simulink model "power_surgnetwork"  (Simulink 6.0)
settings: Solver=ode15s  SolverMode=SingleTasking  StartTime=0.0  StopTime=0.2  RelTol=1e-3  AbsTol=1e-2
libraries: powerlib x21
settings Model: Creator=patrice  LastModifiedBy=batserve  ExtModeTrigMode=oneshot  ExtModeArmWhenConnect=off  ExtModeAutoUpdateStatusClock=off
settings DataIOCC: LimitDataPoints=off  SignalLoggingName=sigsOut
settings OptimizationCC: BlockReduction=off  BooleanDataType=off
settings DebuggingCC: AlgebraicLoopMsg=none  CheckExecutionContextPreStartOutputMsg=on  CheckExecutionContextRuntimeOutputMsg=on  SolverPrmCheckMsg=none
settings HardwareCC: TargetUnknown=on
settings RTWCC: TemplateMakefile=grt_unix.tmf

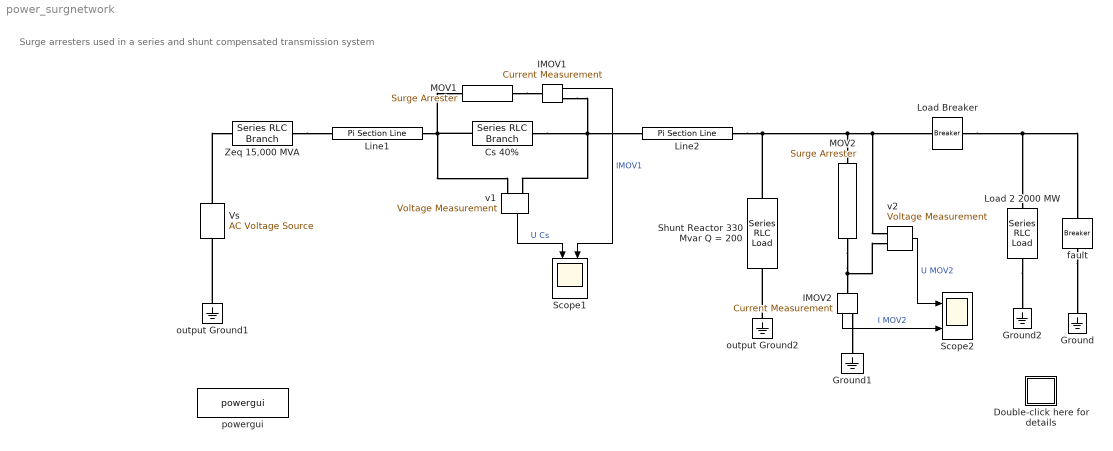
== system power_surgnetwork ==
  note: Surge arresters used in  a series and shunt  compensated
      | transmission system
  Cs 40% : powerlib/Elements/Series RLC Branch  PhysicalDomain=powersysdomain  SubClassName=unknown  LeftPortType=p1  RightPortType=p1  LConnTagsString=__new0  RConnTagsString=__new0  Resistance=0  Inductance=0  Capacitance=101.4e-6  Measurements=None
  Double-click here for details : Subsystem
      mask Display: disp('?')
  Ground : powerlib/Elements/Ground  Orientation=down  PhysicalDomain=powersysdomain  SubClassName=unknown  LeftPortType=p1  RightPortType=p1  LConnTagsString=a
  Ground1 : powerlib/Elements/Ground  Orientation=down  PhysicalDomain=powersysdomain  SubClassName=unknown  LeftPortType=p1  RightPortType=p1  LConnTagsString=a
  Ground2 : powerlib/Elements/Ground  Orientation=down  PhysicalDomain=powersysdomain  SubClassName=unknown  LeftPortType=p1  RightPortType=p1  LConnTagsString=a
  IMOV1 : powerlib/Measurements/Current Measurement  Tag=PoWeRsYsTeMmEaSuReMeNt  PhasorSimulation=off  OutputType=Magnitude  PSBequivalent=0
  IMOV2 : powerlib/Measurements/Current Measurement  Tag=PoWeRsYsTeMmEaSuReMeNt  Orientation=down  PhasorSimulation=off  OutputType=Magnitude  PSBequivalent=0
  Line1 : powerlib/Elements/Pi Section Line  PhysicalDomain=powersysdomain  SubClassName=unknown  LeftPortType=p1  RightPortType=p1  LConnTagsString=__new0  RConnTagsString=__new0  Frequency=60  Resistance=0.011  Inductance=0.8674e-3  Capacitance=13.41e-9  Length=100  PiSections=2  Measurements=None
      settings: AttributesFormatString=\n
  Line2 : powerlib/Elements/Pi Section Line  PhysicalDomain=powersysdomain  SubClassName=unknown  LeftPortType=p1  RightPortType=p1  LConnTagsString=__new0  RConnTagsString=__new0  Frequency=60  Resistance=0.011  Inductance=0.8674e-3  Capacitance=13.41e-9  Length=100  PiSections=2  Measurements=None
      settings: AttributesFormatString=\n
  Load 2 2000 MW : powerlib/Elements/Series RLC Load  Orientation=down  PhysicalDomain=powersysdomain  SubClassName=unknown  LeftPortType=p1  RightPortType=p1  LConnTagsString=a  RConnTagsString=__new0  NominalVoltage=735e3/sqrt(3)  NominalFrequency=60  ActivePower=2000e6/3  InductivePower=0  CapacitivePower=0  Measurements=None
  Load Breaker : powerlib/Elements/Breaker  BreakerResistance=0.1  InitialState=1  SnubberResistance=inf  SnubberCapacitance=0  SwitchingTimes=[ 100e-3]  External=off  Measurements=None
      settings: AttributesFormatString=\n
  MOV1 : powerlib/Elements/Surge Arrester  ProtectionVoltage=185e3  Columns=30  ReferenceCurrent=500  Segment1=[.955 50]  Segment2=[1.0 25]  Segment3=[.9915 16.5]  Measurements=None  MoreParameters=off  BreakLoop=on
      settings: AttributesFormatString=\n
  MOV2 : powerlib/Elements/Surge Arrester  Orientation=down  ProtectionVoltage=1081e3  Columns=2  ReferenceCurrent=500  Segment1=[.955 50]  Segment2=[1.0 25]  Segment3=[.9915 16.5]  Measurements=None  MoreParameters=off  BreakLoop=on
      settings: AttributesFormatString=\n
  Scope1 : Scope  NumInputPorts=2
      settings: Orientation=down  TimeRange=0.2  YMin=-200000~-5000  YMax=200000~10000  DataFormat=Array  MaxDataPoints=500000
  Scope2 : Scope  NumInputPorts=2
      settings: TimeRange=0.2  YMin=-2e+006~0  YMax=2e+006~1000  DataFormat=Array  MaxDataPoints=500000
  Shunt Reactor 330 Mvar Q = 200 : powerlib/Elements/Series RLC Load  Orientation=up  PhysicalDomain=powersysdomain  SubClassName=unknown  LeftPortType=p1  RightPortType=p1  LConnTagsString=a  RConnTagsString=__new0  NominalVoltage=735e3/sqrt(3)  NominalFrequency=60  ActivePower=330e6/3/200  InductivePower=330e6/3  CapacitivePower=0  Measurements=None
  Vs : powerlib/Electrical Sources/AC Voltage Source  Description=source block  Orientation=up  Amplitude=735e3/sqrt(3)*sqrt(2)  Phase=0  Frequency=60  SampleTime=0  Measurements=None
      settings: AttributesFormatString=\n
  Zeq 15,000 MVA : powerlib/Elements/Series RLC Branch  PhysicalDomain=powersysdomain  SubClassName=unknown  LeftPortType=p1  RightPortType=p1  LConnTagsString=__new0  RConnTagsString=__new0  Resistance=3.6  Inductance=95.5e-3  Capacitance=inf  Measurements=None
  fault : powerlib/Elements/Breaker  Orientation=down  BreakerResistance=1  InitialState=0  SnubberResistance=inf  SnubberCapacitance=0  SwitchingTimes=[ 30e-3 300e-3]  External=off  Measurements=None
      settings: AttributesFormatString=\n
  output Ground1 : powerlib/Elements/Ground  Orientation=down  PhysicalDomain=powersysdomain  SubClassName=unknown  LeftPortType=p1  RightPortType=p1  LConnTagsString=a
  output Ground2 : powerlib/Elements/Ground  Orientation=down  PhysicalDomain=powersysdomain  SubClassName=unknown  LeftPortType=p1  RightPortType=p1  LConnTagsString=a
  powergui : powerlib/powergui  Priority=2  Frange=logspace(0,3,50)  Ylog=off  Xlog=off  save=off  variable=ZData  ZoomFFT=on  StartTime=0.0  cycles=1  DisplayStyle=off  fundamental=60  FreqAxis=off  MaxFrequency=1000  frequencyindice=1  frequencyindicesteady=1  RmsSteady=1  display=off  Ts=0  methode=off  frequency=60  echomessages=on
  v1 : powerlib/Measurements/Voltage Measurement  Tag=PoWeRsYsTeMmEaSuReMeNt  Orientation=down  PhasorSimulation=off  OutputType=Magnitude  PSBequivalent=0
  v2 : powerlib/Measurements/Voltage Measurement  Tag=PoWeRsYsTeMmEaSuReMeNt  PhasorSimulation=off  OutputType=Magnitude  PSBequivalent=0
  wires:
  v2/1 -> Scope2/1  "U MOV2"
  IMOV2/1 -> Scope2/2  "I MOV2"
  v1/1 -> Scope1/1  "U Cs"
  IMOV1/1 -> Scope1/2  "IMOV1"
  connections:
  output Ground1/LConn1 -- Vs/LConn1
  Vs/RConn1 -- Zeq 15,000 MVA/LConn1
  Zeq 15,000 MVA/RConn1 -- Line1/LConn1
  MOV1/RConn1 -- IMOV1/LConn1
  Cs 40%/LConn1 -- Line1/RConn1 -- MOV1/LConn1 -- v1/LConn1
  Cs 40%/RConn1 -- Line2/LConn1 -- IMOV1/RConn1 -- v1/LConn2
  output Ground2/LConn1 -- Shunt Reactor 330 Mvar Q = 200/LConn1
  fault/RConn1 -- Ground/LConn1
  Load 2 2000 MW/RConn1 -- Ground2/LConn1
  Load Breaker/RConn1 -- Load 2 2000 MW/LConn1 -- fault/LConn1
  MOV2/RConn1 -- IMOV2/LConn1 -- v2/LConn2
  IMOV2/RConn1 -- Ground1/LConn1
  Line2/RConn1 -- MOV2/LConn1 -- Load Breaker/LConn1 -- v2/LConn1 -- Shunt Reactor 330 Mvar Q = 200/RConn1

== system power_surgnetwork/Double-click here for details ==
  note: Start the simulation.  Observe the MOV voltages and currents on Scope1 and Scope2.
      |
      | At fault application  the capacitor voltage increases and  MOV1 conducts. Peak current  reaches  8.4 kA on the 2nd pulse
      | 2 cycles after fault application,  the MOV current is symetric  (4.5 kA current pulses at every half cycle).
      |
      | At fault clearing, the  overvoltage  produced at bus B2 is limited by the shunt MOV2 .
      | The fast transient produces a 850 A current pulse in the MOV.
  note: A 735 kV equivalent transmission systems feeds a load through a 200 km transmission line. The line is series compensated at the
      | middle point and shunt compensated at its receiving end.  A fault  is applied at the load terminals.
      | The fault is cleared by load breaker opening. For simplification purpose, only  one phase of the transmission system is modelled.
      | All parameters correspond to positive-sequence.
      |
      | The  three-phase  short circuit level of the transmission system is 15000 MVA. The line is 40% series compensated by a capacitor
      | (26.2 ohms at 60 Hz) and shunt compensated by a 330 Mvar (110 Mvar/phase) inductor  at the load end.
      |
      | The series capacitor and shunt inductor are both protected by metal oxide varistors (MOV).
      | The series capacitor  varistor  MOV1 consists of 30 columns protecting the capacitor at 2.5 times
      | its rated voltage (rated voltage is obtained for a 2000 kA line rated current).
      | The corresponding protection  voltage (defined at 15 kA = 500 A per column) is 2.5*26.2 *2kA*sqrt(2) = 185 kV.
      |
      | The shunt inductor is protected by a 2-column arrester  (MOV2) at 1.8 p.u. of nominal
      | phase-to-ground voltage (424.4 kVrms). The corresponding protection voltage (defined at 1 kA or 500A /column)
      | is 1.8*424.4*sqrt(2) = 1080 kV.
  note: This demonstration illustrates use of surge arresters in a
      | series and shunt compensated 735 kV AC transmission system
  note: Circuit Description
  note: Demonstration
  note: G. Sybille (Hydro-Quebec)
